simulink model "quarterCar"  (R2017b)
settings: Solver=VariableStepAuto  StartTime=0.0  StopTime=10.0  RelTol=1e-3
libraries: simulink x1
settings Model: Creator=cs756  LastModifiedBy=cs756

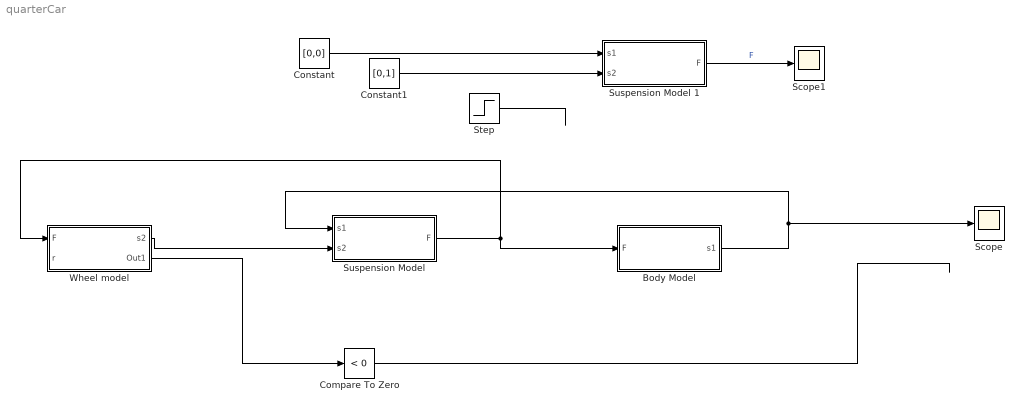
== system quarterCar ==
  Body Model : Subsystem  mask{m1=250, g=9.81}
      mask prompts: m1 "Body Mass"
  Compare To Zero : simulink/Logic and Bit Operations/Compare To Zero  relop=<  OutDataTypeStr=boolean
  Constant : Constant  Value=[0,0]
  Constant1 : Constant  Value=[0,1]
  Scope : Scope
  Scope1 : Scope
  Step : Step  SampleTime=0
  "Suspension Model " : Subsystem  mask{cs1=1000, cs2=1000, ks=20000, ks2=20000, x0=2, x1=2}
      mask prompts: cs1 "Damper Compression coefficient"; cs2 "Damper Tension coefficient"; ks "Stiffness coefficient"; ks2 "Stiffness addition"; x0 "Elastic spring extension limit"; x1 "Damper motion range"
  Suspension Model 1 : Subsystem  mask{cs1=1000, cs2=2000, ks=20000, ks2=10000, x0=2, x1=2}
      mask prompts: cs1 "Damper Compression coefficient"; cs2 "Damper Tension coefficient"; ks "Stiffness coefficient"; ks2 "Stiffness addition"; x0 "Elastic spring extension limit"; x1 "Damper motion range"
  "Wheel model " : Subsystem  mask{kt=140000, kt2=140000, m2=20, g=9.81, x0=1}
      mask prompts: kt "Wheel soft stiffness"; kt2 "Wheel hard stiffness"; m2 "Wheel mass"; x0 "Wheel elastic extension limit"
  wires:
  Body Model/1(s1) -> Scope/1, "Suspension Model "/1(s1)
  "Suspension Model "/1(F) -> Body Model/1(F), "Wheel model "/1(F)
  "Wheel model "/1(s2) -> "Suspension Model "/2(s2)
  Step/1 -> ?
  "Wheel model "/2(Out1) -> Compare To Zero/1
  Compare To Zero/1 -> ?
  Constant1/1 -> Suspension Model 1/2(s2)
  Constant/1 -> Suspension Model 1/1(s1)
  Suspension Model 1/1(F) -> Scope1/1  "F"

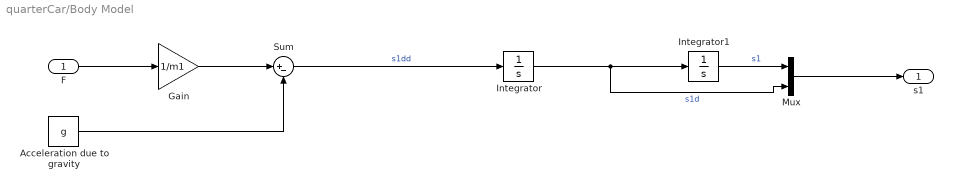
== system quarterCar/Body Model ==
  F : Inport
  Acceleration due to gravity : Constant  Value=g
  Gain : Gain  Gain=1/m1
  Integrator : Integrator
  Integrator1 : Integrator
  Mux : Mux  Inputs=2
  Sum : Sum  Inputs=|+-
  s1 : Outport
  wires:
  Acceleration due to gravity/1 -> Sum/2
  Sum/1 -> Integrator/1  "s1dd"
  Integrator/1 -> Mux/2, Integrator1/1  "s1d"
  F/1 -> Gain/1
  Gain/1 -> Sum/1
  Mux/1 -> s1/1
  Integrator1/1 -> Mux/1  "s1"

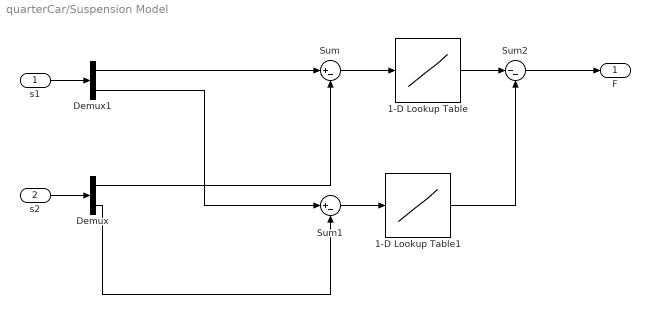
== system quarterCar/Suspension Model  ==
  s1 : Inport
  s2 : Inport  Port=2
  1-D Lookup Table : Lookup_n-D  NumberOfTableDimensions=1  BreakpointsForDimension1=[-2*x0, -x0, x0, 2*x0]  Table=[-(ks+ks2)*x0,-ks*x0,ks*x0,(ks+ks2)*x0]  InternalRulePriority=Speed  RndMeth=Simplest  InputSameDT=on
  1-D Lookup Table1 : Lookup_n-D  NumberOfTableDimensions=1  BreakpointsForDimension1=[-x1, 0, x1]  Table=[-cs2*x1, 0, cs1*x1]  InternalRulePriority=Speed  RndMeth=Simplest  InputSameDT=on
  Demux : Demux  Outputs=2
  Demux1 : Demux  Outputs=2
  Sum : Sum  Inputs=|+-
  Sum1 : Sum  Inputs=|+-
  Sum2 : Sum  Inputs=|--
  F : Outport
  wires:
  Sum/1 -> 1-D Lookup Table/1
  Sum2/1 -> F/1
  s2/1 -> Demux/1
  Demux/1 -> Sum/2
  Demux/2 -> Sum1/2
  Demux1/1 -> Sum/1
  s1/1 -> Demux1/1
  Demux1/2 -> Sum1/1
  1-D Lookup Table/1 -> Sum2/1
  Sum1/1 -> 1-D Lookup Table1/1
  1-D Lookup Table1/1 -> Sum2/2

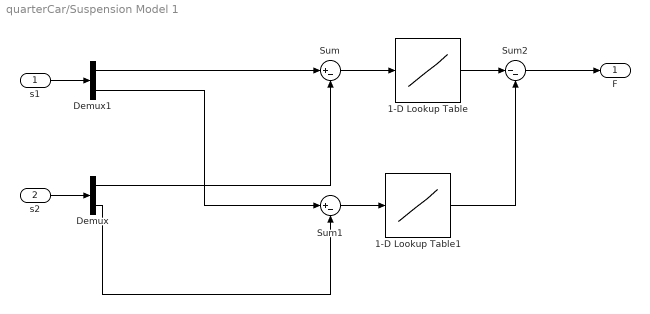
== system quarterCar/Suspension Model 1 ==
  s1 : Inport
  s2 : Inport  Port=2
  1-D Lookup Table : Lookup_n-D  NumberOfTableDimensions=1  BreakpointsForDimension1=[-2*x0, -x0, x0, 2*x0]  Table=[-(ks+ks2)*x0,-ks*x0,ks*x0,(ks+ks2)*x0]  InternalRulePriority=Speed  RndMeth=Simplest  InputSameDT=on
  1-D Lookup Table1 : Lookup_n-D  NumberOfTableDimensions=1  BreakpointsForDimension1=[-x1, 0, x1]  Table=[-cs2*x1, 0, cs1*x1]  InternalRulePriority=Speed  RndMeth=Simplest  InputSameDT=on
  Demux : Demux  Outputs=2
  Demux1 : Demux  Outputs=2
  Sum : Sum  Inputs=|+-
  Sum1 : Sum  Inputs=|+-
  Sum2 : Sum  Inputs=|--
  F : Outport
  wires:
  Sum/1 -> 1-D Lookup Table/1
  Sum2/1 -> F/1
  s2/1 -> Demux/1
  Demux/1 -> Sum/2
  Demux/2 -> Sum1/2
  Demux1/1 -> Sum/1
  s1/1 -> Demux1/1
  Demux1/2 -> Sum1/1
  1-D Lookup Table/1 -> Sum2/1
  Sum1/1 -> 1-D Lookup Table1/1
  1-D Lookup Table1/1 -> Sum2/2

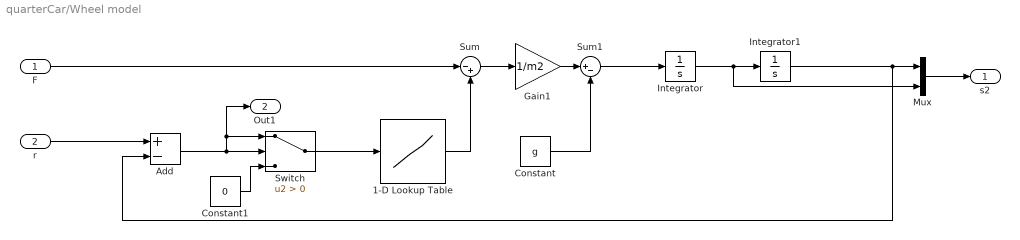
== system quarterCar/Wheel model  ==
  F : Inport
  r : Inport  Port=2
  1-D Lookup Table : Lookup_n-D  NumberOfTableDimensions=1  BreakpointsForDimension1=[-2*x0, -x0, x0, 2*x0]  Table=[-(kt+kt2)*x0,-kt*x0,kt*x0,(kt+kt2)*x0]  InternalRulePriority=Speed  RndMeth=Simplest  InputSameDT=on
  Add : Sum  Inputs=+-
  Constant : Constant  Value=g
  Constant1 : Constant  Value=0
  Gain1 : Gain  Gain=1/m2
  Integrator : Integrator
  Integrator1 : Integrator
  Mux : Mux  Inputs=2
  Sum : Sum  Inputs=|-+
  Sum1 : Sum  Inputs=|+-
  Switch : Switch  Criteria=u2 > Threshold
  s2 : Outport
  Out1 : Outport  Port=2
  wires:
  r/1 -> Add/1
  F/1 -> Sum/1
  Add/1 -> Out1/1, Switch/1, Switch/2
  Constant1/1 -> Switch/3
  Switch/1 -> 1-D Lookup Table/1
  1-D Lookup Table/1 -> Sum/2
  Sum/1 -> Gain1/1
  Gain1/1 -> Sum1/1
  Constant/1 -> Sum1/2
  Sum1/1 -> Integrator/1
  Integrator/1 -> Mux/2, Integrator1/1
  Integrator1/1 -> Add/2, Mux/1
  Mux/1 -> s2/1
